simulink library "typhoonPatterns"  (R2017b)
settings: Solver=VariableStepAuto  StartTime=0.0  StopTime=10.0  RelTol=1e-3
undefined symbols (not defined in the file or in its folder): c_clamp, C_l, c_picoup_seq, crun_sp_ind, cst_sp_ind, f, f_picoup, f_sp_ind, fc, Jm, L, L1, L2, L_l, l_picoup_seq, La_DC, Ld, Lf_DC, Llr1_ind, Llr2_ind, Llr_ind, llrm_sp_ind, Lls_ind, llsa_sp_ind, llsm_sp_ind, Lm, Lq, n1, n2, nanm_sp_ind, pms, R, R1, R2, r_clamp, R_l, r_picoup_seq, Ra_DC, Rf_DC, Rm, Rr1_ind, Rr2_ind, Rr_ind, rrm_sp_ind, rrun_sp_ind, Rs, Rs_ind, rsa_sp_ind, rsm_sp_ind, rst_sp_ind
libraries: powerlib x282
(part 1 of 3)
settings Model: Creator=marco  LastModifiedBy=Marcos

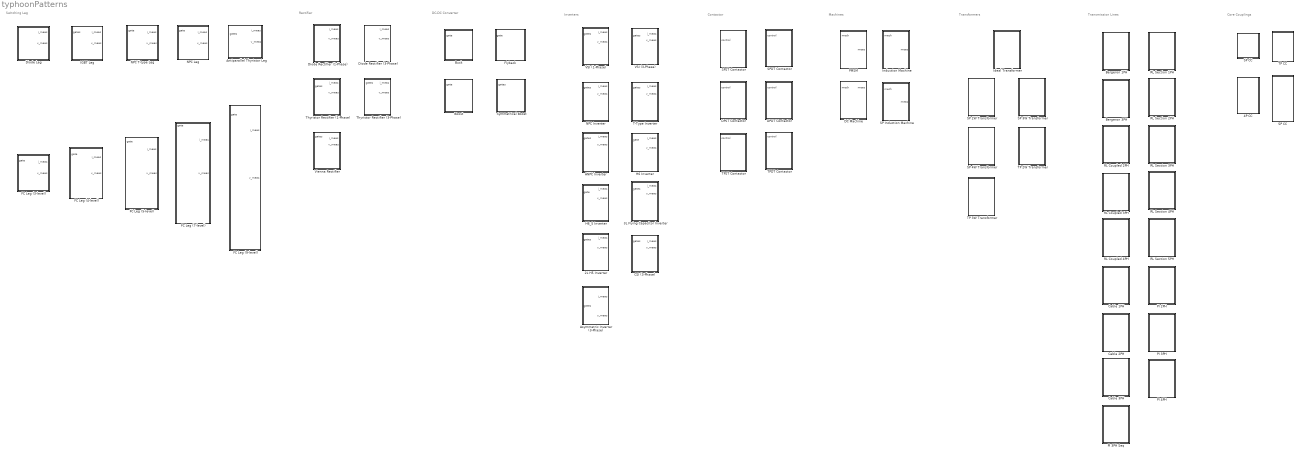
== system typhoonPatterns ==
  note: Rectifier
  note: Switching Leg
  note: DC-DC Converter
  note: Contactor
  note: Inverters
  note: Machines
  note: Transformers
  note: Transmission Lines
  note: Core Couplings
  2L H5 Inverter : Subsystem
  3L Flying Capacitor Inverter : Subsystem
  4P CC : Subsystem
  5P CC : Subsystem
  ANPC Inverter : Subsystem
  Antiparallel Thyristor Leg : Subsystem
  Asymmetric Inverter (3-Phase) : Subsystem
  Bergeron 1PH : Subsystem
  Bergeron 3PH : Subsystem
  Boost : Subsystem
  Buck : Subsystem
  CSI (3-Phase) : Subsystem
  Cable 1PH : Subsystem
  Cable 2PH : Subsystem
  Cable 3PH : Subsystem
  DC Machine : Subsystem
  DPDT Contactor : Subsystem
  DPST Contactor : Subsystem
  Diode Leg : Subsystem
  Diode Rectifier (1-Phase) : Subsystem
  Diode Rectifier (3-Phase) : Subsystem
  FC Leg (3-level) : Subsystem
  FC Leg (4-level) : Subsystem
  FC Leg (5-level) : Subsystem
  FC Leg (7-level) : Subsystem
  FC Leg (9-level) : Subsystem
  Flyback : Subsystem
  H6 Inverter : Subsystem
  H6_5 Inverter : Subsystem
  IGBT Leg : Subsystem
  Ideal Transformer : Subsystem
  Induction Machine : Subsystem
  NPC Inverter : Subsystem
  NPC Leg : Subsystem
  NPC T-type Leg : Subsystem
  PI 2PH : Subsystem
  PI 3PH : Subsystem
  PI 3PH Seq : Subsystem
  PI 4PH : Subsystem
  PMSM : Subsystem
  RL Coupled 2PH : Subsystem
  RL Coupled 3PH : Subsystem
  RL Coupled 4PH : Subsystem
  RL Section 1PH : Subsystem
  RL Section 2PH : Subsystem
  RL Section 3PH : Subsystem
  RL Section 4PH : Subsystem
  RL Section 5PH : Subsystem
  SP 2W Transformer : Subsystem
  SP 3W Transformer : Subsystem
  SP 4W Transformer : Subsystem
  SP CC : Subsystem
  SP Induction Machine : Subsystem
  SPDT Contactor : Subsystem
  SPST Contactor : Subsystem
  Symmetrical Boost : Subsystem
  T-Type Inverter : Subsystem
  TP 2W Transformer : Subsystem
  TP 3W Transformer : Subsystem
  TP CC : Subsystem
  TPDT Contactor : Subsystem
  TPST Contactor : Subsystem
  Thyristor Rectifier (1-Phase) : Subsystem
  Thyristor Rectifier (3-Phase) : Subsystem
  VSI (1-Phase) : Subsystem
  VSI (3-Phase) : Subsystem
  Vienna Rectifier : Subsystem

== system typhoonPatterns/2L H5 Inverter ==
  gates : Inport
  Bus Creator : BusCreator  Inputs=5
  Bus Creator1 : BusCreator  Inputs=5
  Demux{1..3,5..6} (5 alike) : Demux  Outputs=2
  Demux4 : Demux  Outputs=5
  S5 : powerlib/Power Electronics/IGBT//Diode  Ron=r_on  Rs=r_s  Cs=c_s  Measurements=on
  Selector_i : BusSelector  OutputSignals=i(Sa_top)  OutputAsBus=on
  Selector_v : BusSelector  OutputSignals=v(Sa_top)  OutputAsBus=on
  inv{1..5} (5 alike) : Logic  Commented=through  Operator=NOT  AllPortsSameDT=off  OutDataTypeStr=boolean
  sa_bot : powerlib/Power Electronics/IGBT//Diode  Ron=r_on  Rs=r_s  Cs=c_s  Measurements=on
  sa_top : powerlib/Power Electronics/IGBT//Diode  Ron=r_on  Rs=r_s  Cs=c_s  Measurements=on
  sb_bot : powerlib/Power Electronics/IGBT//Diode  Ron=r_on  Rs=r_s  Cs=c_s  Measurements=on
  sb_top : powerlib/Power Electronics/IGBT//Diode  Ron=r_on  Rs=r_s  Cs=c_s  Measurements=on
  A : PMIOPort  Port=1  Side=Right
  B : PMIOPort  Port=2  Side=Right
  DC+ : PMIOPort  Port=3  Side=Left
  DC- : PMIOPort  Port=4  Side=Left
  i_meas : Outport
  v_meas : Outport  Port=2
  wires:
  sb_top/1 -> [m_Sb_top]
  sa_top/1 -> [m_Sa_top]
  [Sb_top] -> sb_top/1
  sb_bot/1 -> [m_Sb_bot]
  [Sa_top] -> sa_top/1
  [Sb_bot] -> sb_bot/1
  sa_bot/1 -> [m_Sa_bot]
  [Sa_bot] -> sa_bot/1
  inv4/1 -> [Sb_bot]
  Demux4/4 -> inv4/1
  Demux4/2 -> inv2/1
  inv2/1 -> [Sa_bot]
  gates/1 -> Demux4/1
  inv3/1 -> [Sb_top]
  Demux4/3 -> inv3/1
  inv1/1 -> [Sa_top]
  Demux4/1 -> inv1/1
  Demux2/2 -> [v_Sa_bot]
  Demux1/2 -> [v_Sa_top]
  [v_Sa_top] -> Bus Creator1/1  "v(Sa_top)"
  [i_Sb_top] -> Bus Creator/3  "i(Sb_top)"
  [i_Sb_bot] -> Bus Creator/4  "i(Sb_bot)"
  Demux5/2 -> [v_Sb_bot]
  Bus Creator1/1 -> Selector_v/1
  Demux3/2 -> [v_Sb_top]
  [v_Sb_bot] -> Bus Creator1/4  "v(Sb_bot)"
  Demux5/1 -> [i_Sb_bot]
  Selector_v/1 -> v_meas/1
  [v_Sb_top] -> Bus Creator1/3  "v(Sb_top)"
  [m_Sb_bot] -> Demux5/1
  [m_Sa_bot] -> Demux2/1
  Demux1/1 -> [i_Sa_top]
  [m_Sa_top] -> Demux1/1
  Bus Creator/1 -> Selector_i/1
  [m_Sb_top] -> Demux3/1
  Demux2/1 -> [i_Sa_bot]
  Selector_i/1 -> i_meas/1
  Demux3/1 -> [i_Sb_top]
  [v_Sa_bot] -> Bus Creator1/2  "v(Sa_bot)"
  [i_Sa_bot] -> Bus Creator/2  "i(Sa_bot)"
  [i_Sa_top] -> Bus Creator/1  "i(Sa_top)"
  inv5/1 -> [S5]
  Demux4/5 -> inv5/1
  [S5] -> S5/1
  S5/1 -> [m_S5]
  [m_S5] -> Demux6/1
  Demux6/1 -> [i_S5]
  Demux6/2 -> [v_S5]
  [v_S5] -> Bus Creator1/5  "v(S5)"
  [i_S5] -> Bus Creator/5  "i(S5)"
  connections:
  sa_top/LConn1 -- sa_bot/RConn1 -- A/RConn1
  sb_top/LConn1 -- sb_bot/RConn1 -- B/RConn1
  sa_bot/LConn1 -- sb_bot/LConn1 -- DC-/RConn1
  sb_top/RConn1 -- S5/RConn1 -- sa_top/RConn1
  DC+/RConn1 -- S5/LConn1

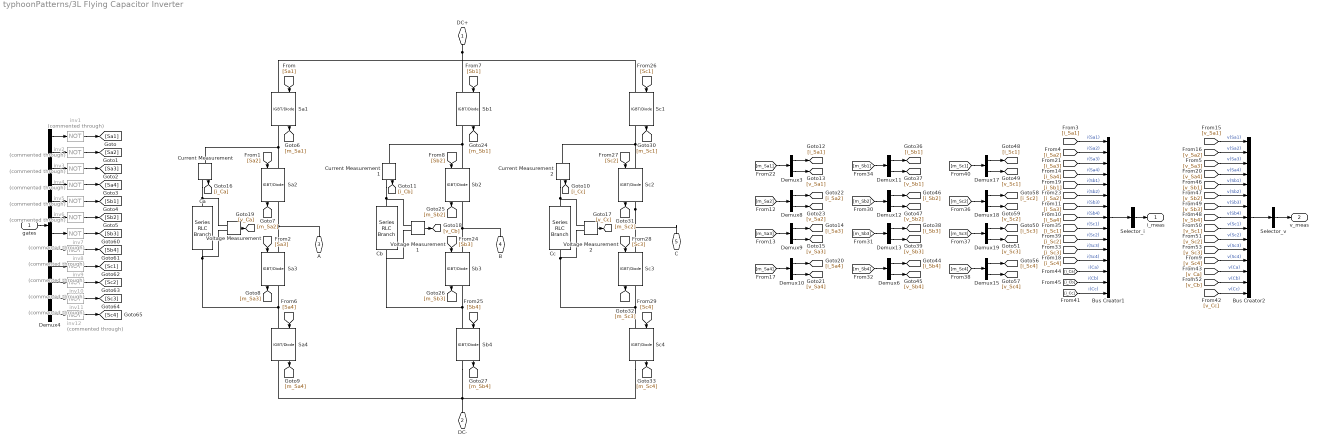
== system typhoonPatterns/3L Flying Capacitor Inverter ==
  gates : Inport
  Bus Creator1 : BusCreator  Inputs=15
  Bus Creator2 : BusCreator  Inputs=15
  Ca : powerlib/Elements/Series RLC Branch  LConnTagsString=__new0  RConnTagsString=__new0  BranchType=RC  Resistance=r_clamp  Inductance=1e-3  SetiL0=off  InitialCurrent=0  Capacitance=c_clamp  Setx0=on  InitialVoltage=v0_clamp  Measurements=None
  Cb : powerlib/Elements/Series RLC Branch  LConnTagsString=__new0  RConnTagsString=__new0  BranchType=RC  Resistance=r_clamp  Inductance=1e-3  SetiL0=off  InitialCurrent=0  Capacitance=c_clamp  Setx0=on  InitialVoltage=v0_clamp  Measurements=None
  Cc : powerlib/Elements/Series RLC Branch  LConnTagsString=__new0  RConnTagsString=__new0  BranchType=RC  Resistance=r_clamp  Inductance=1e-3  SetiL0=off  InitialCurrent=0  Capacitance=c_clamp  Setx0=on  InitialVoltage=v0_clamp  Measurements=None
  Current Measurement : powerlib/Measurements/Current Measurement  PhasorSimulation=off  OutputType=Complex  PSBequivalent=0
  Current Measurement1 : powerlib/Measurements/Current Measurement  PhasorSimulation=off  OutputType=Complex  PSBequivalent=0
  Current Measurement2 : powerlib/Measurements/Current Measurement  PhasorSimulation=off  OutputType=Complex  PSBequivalent=0
  Demux{3,6,8..13,15,17..19} (12 alike) : Demux  Outputs=2
  Demux4 : Demux  Outputs=12
  Sa{1..4} (4 alike) : powerlib/Power Electronics/IGBT//Diode  Ron=r_on  Rs=r_s  Cs=c_s  Measurements=on
  Sb{1..4} (4 alike) : powerlib/Power Electronics/IGBT//Diode  Ron=r_on  Rs=r_s  Cs=c_s  Measurements=on
  Sc{1..4} (4 alike) : powerlib/Power Electronics/IGBT//Diode  Ron=r_on  Rs=r_s  Cs=c_s  Measurements=on
  Selector_i : BusSelector  OutputSignals=i(Sa1)  OutputAsBus=on
  Selector_v : BusSelector  OutputSignals=v(Sa1)  OutputAsBus=on
  Voltage Measurement : powerlib/Measurements/Voltage Measurement  PhasorSimulation=off  OutputType=Complex  PSBequivalent=0
  Voltage Measurement1 : powerlib/Measurements/Voltage Measurement  PhasorSimulation=off  OutputType=Complex  PSBequivalent=0
  Voltage Measurement2 : powerlib/Measurements/Voltage Measurement  PhasorSimulation=off  OutputType=Complex  PSBequivalent=0
  inv{1..12} (12 alike) : Logic  Commented=through  Operator=NOT  AllPortsSameDT=off  OutDataTypeStr=boolean
  DC+ : PMIOPort  Port=1  Side=Left
  DC- : PMIOPort  Port=2  Side=Left
  A : PMIOPort  Port=3  Side=Right
  B : PMIOPort  Port=4  Side=Right
  C : PMIOPort  Port=5  Side=Right
  i_meas : Outport
  v_meas : Outport  Port=2
  wires:
  inv9/1 -> [Sc1]
  Demux4/7 -> inv7/1
  Demux4/11 -> inv11/1
  Demux4/9 -> inv9/1
  Demux4/8 -> inv8/1
  inv7/1 -> [Sb3]
  inv10/1 -> [Sc2]
  inv12/1 -> [Sc4]
  inv11/1 -> [Sc3]
  Demux4/10 -> inv10/1
  inv8/1 -> [Sb4]
  Demux4/12 -> inv12/1
  Demux17/1 -> [i_Sc1]
  Demux15/1 -> [i_Sc4]
  [m_Sc2] -> Demux18/1
  [m_Sc1] -> Demux17/1
  Demux19/1 -> [i_Sc3]
  Demux19/2 -> [v_Sc3]
  Demux17/2 -> [v_Sc1]
  Demux18/2 -> [v_Sc2]
  [m_Sc4] -> Demux15/1
  Demux15/2 -> [v_Sc4]
  Demux18/1 -> [i_Sc2]
  [m_Sc3] -> Demux19/1
  Demux11/1 -> [i_Sb1]
  Demux6/1 -> [i_Sb4]
  [m_Sb2] -> Demux12/1
  [m_Sb1] -> Demux11/1
  Demux13/1 -> [i_Sb3]
  Demux13/2 -> [v_Sb3]
  Demux11/2 -> [v_Sb1]
  Demux12/2 -> [v_Sb2]
  [m_Sb4] -> Demux6/1
  Demux6/2 -> [v_Sb4]
  Demux12/1 -> [i_Sb2]
  [m_Sb3] -> Demux13/1
  [Sc2] -> Sc2/1
  Sc1/1 -> [m_Sc1]
  Sc4/1 -> [m_Sc4]
  Sc2/1 -> [m_Sc2]
  [Sc1] -> Sc1/1
  Sc3/1 -> [m_Sc3]
  [Sc3] -> Sc3/1
  [Sc4] -> Sc4/1
  [Sb2] -> Sb2/1
  Sb1/1 -> [m_Sb1]
  Sb4/1 -> [m_Sb4]
  Sb2/1 -> [m_Sb2]
  [Sb1] -> Sb1/1
  Sb3/1 -> [m_Sb3]
  [Sb3] -> Sb3/1
  [Sb4] -> Sb4/1
  [Sa2] -> Sa2/1
  Sa1/1 -> [m_Sa1]
  Sa4/1 -> [m_Sa4]
  Sa2/1 -> [m_Sa2]
  [Sa1] -> Sa1/1
  Sa3/1 -> [m_Sa3]
  [Sa3] -> Sa3/1
  [Sa4] -> Sa4/1
  Selector_v/1 -> v_meas/1
  Demux3/1 -> [i_Sa1]
  Demux4/3 -> inv3/1
  [v_Sa4] -> Bus Creator2/4  "v(Sa4)"
  [v_Sa3] -> Bus Creator2/3  "v(Sa3)"
  inv4/1 -> [Sa4]
  [i_Sa4] -> Bus Creator1/4  "i(Sa4)"
  Demux3/2 -> [v_Sa1]
  inv2/1 -> [Sa2]
  inv1/1 -> [Sa1]
  inv5/1 -> [Sb1]
  inv3/1 -> [Sa3]
  gates/1 -> Demux4/1
  inv6/1 -> [Sb2]
  Demux4/1 -> inv1/1
  Demux4/6 -> inv6/1
  Demux8/1 -> [i_Sa2]
  Bus Creator2/1 -> Selector_v/1
  [i_Sa1] -> Bus Creator1/1  "i(Sa1)"
  Demux9/2 -> [v_Sa3]
  Demux9/1 -> [i_Sa3]
  [v_Sa1] -> Bus Creator2/1  "v(Sa1)"
  Demux8/2 -> [v_Sa2]
  [i_Sa3] -> Bus Creator1/3  "i(Sa3)"
  Demux4/5 -> inv5/1
  Demux10/2 -> [v_Sa4]
  Demux4/4 -> inv4/1
  [m_Sa2] -> Demux8/1
  [m_Sa3] -> Demux9/1
  [m_Sa4] -> Demux10/1
  Demux10/1 -> [i_Sa4]
  Bus Creator1/1 -> Selector_i/1
  [v_Sa2] -> Bus Creator2/2  "v(Sa2)"
  Selector_i/1 -> i_meas/1
  Demux4/2 -> inv2/1
  [m_Sa1] -> Demux3/1
  [i_Sa2] -> Bus Creator1/2  "i(Sa2)"
  Current Measurement/1 -> [i_Ca]
  Current Measurement1/1 -> [i_Cb]
  Current Measurement2/1 -> [i_Cc]
  Voltage Measurement/1 -> [v_Ca]
  Voltage Measurement2/1 -> [v_Cc]
  Voltage Measurement1/1 -> [v_Cb]
  [i_Cb] -> Bus Creator1/14  "i(Cb)"
  [i_Ca] -> Bus Creator1/13  "i(Ca)"
  [i_Cc] -> Bus Creator1/15  "i(Cc)"
  [i_Sa2] -> Bus Creator1/6  "i(Sb2)"
  [i_Sa3] -> Bus Creator1/7  "i(Sb3)"
  [i_Sb1] -> Bus Creator1/5  "i(Sb1)"
  [i_Sa4] -> Bus Creator1/8  "i(Sb4)"
  [i_Sc4] -> Bus Creator1/12  "i(Sc4)"
  [i_Sc3] -> Bus Creator1/11  "i(Sc3)"
  [i_Sc2] -> Bus Creator1/10  "i(Sc2)"
  [i_Sc1] -> Bus Creator1/9  "i(Sc1)"
  [v_Ca] -> Bus Creator2/13  "v(Ca)"
  [v_Cb] -> Bus Creator2/14  "v(Cb)"
  [v_Cc] -> Bus Creator2/15  "v(Cc)"
  [v_Sb3] -> Bus Creator2/7  "v(Sb3)"
  [v_Sb2] -> Bus Creator2/6  "v(Sb2)"
  [v_Sb1] -> Bus Creator2/5  "v(Sb1)"
  [v_Sb4] -> Bus Creator2/8  "v(Sb4)"
  [v_Sc3] -> Bus Creator2/11  "v(Sc3)"
  [v_Sc4] -> Bus Creator2/12  "v(Sc4)"
  [v_Sc2] -> Bus Creator2/10  "v(Sc2)"
  [v_Sc1] -> Bus Creator2/9  "v(Sc1)"
  connections:
  Sc2/LConn1 -- Current Measurement2/LConn1 -- Sc1/RConn1
  Sc4/LConn1 -- Voltage Measurement2/LConn2 -- Cc/RConn1 -- Sc3/RConn1
  Sc2/RConn1 -- Sc3/LConn1 -- C/RConn1
  Sb2/LConn1 -- Current Measurement1/LConn1 -- Sb1/RConn1
  Sb4/LConn1 -- Voltage Measurement1/LConn2 -- Cb/RConn1 -- Sb3/RConn1
  Sb3/LConn1 -- B/RConn1 -- Sb2/RConn1
  Sc4/RConn1 -- Sb4/RConn1 -- Sa4/RConn1 -- DC-/RConn1
  DC+/RConn1 -- Sb1/LConn1 -- Sc1/LConn1 -- Sa1/LConn1
  Ca/LConn1 -- Current Measurement/RConn1 -- Voltage Measurement/LConn1
  Sa4/LConn1 -- Voltage Measurement/LConn2 -- Ca/RConn1 -- Sa3/RConn1
  Sa3/LConn1 -- A/RConn1 -- Sa2/RConn1
  Sa2/LConn1 -- Current Measurement/LConn1 -- Sa1/RConn1
  Current Measurement1/RConn1 -- Voltage Measurement1/LConn1 -- Cb/LConn1
  Current Measurement2/RConn1 -- Voltage Measurement2/LConn1 -- Cc/LConn1

== system typhoonPatterns/4P CC ==
  a_in : PMIOPort  Port=1  Side=Left
  b_in : PMIOPort  Port=2  Side=Left
  a_out : PMIOPort  Port=3  Side=Right
  b_out : PMIOPort  Port=4  Side=Right
  c_in : PMIOPort  Port=5  Side=Left
  c_out : PMIOPort  Port=6  Side=Right
  d_in : PMIOPort  Port=7  Side=Left
  d_out : PMIOPort  Port=8  Side=Right
  connections:
  c_in/RConn1 -- c_out/RConn1
  b_in/RConn1 -- b_out/RConn1
  a_in/RConn1 -- a_out/RConn1
  d_in/RConn1 -- d_out/RConn1

== system typhoonPatterns/5P CC ==
  a_in : PMIOPort  Port=1  Side=Left
  b_in : PMIOPort  Port=2  Side=Left
  a_out : PMIOPort  Port=3  Side=Right
  b_out : PMIOPort  Port=4  Side=Right
  c_in : PMIOPort  Port=5  Side=Left
  c_out : PMIOPort  Port=6  Side=Right
  d_in : PMIOPort  Port=7  Side=Left
  d_out : PMIOPort  Port=8  Side=Right
  e_in : PMIOPort  Port=9  Side=Left
  e_out : PMIOPort  Port=10  Side=Right
  connections:
  c_in/RConn1 -- c_out/RConn1
  a_in/RConn1 -- a_out/RConn1
  b_in/RConn1 -- b_out/RConn1
  d_in/RConn1 -- d_out/RConn1
  e_in/RConn1 -- e_out/RConn1

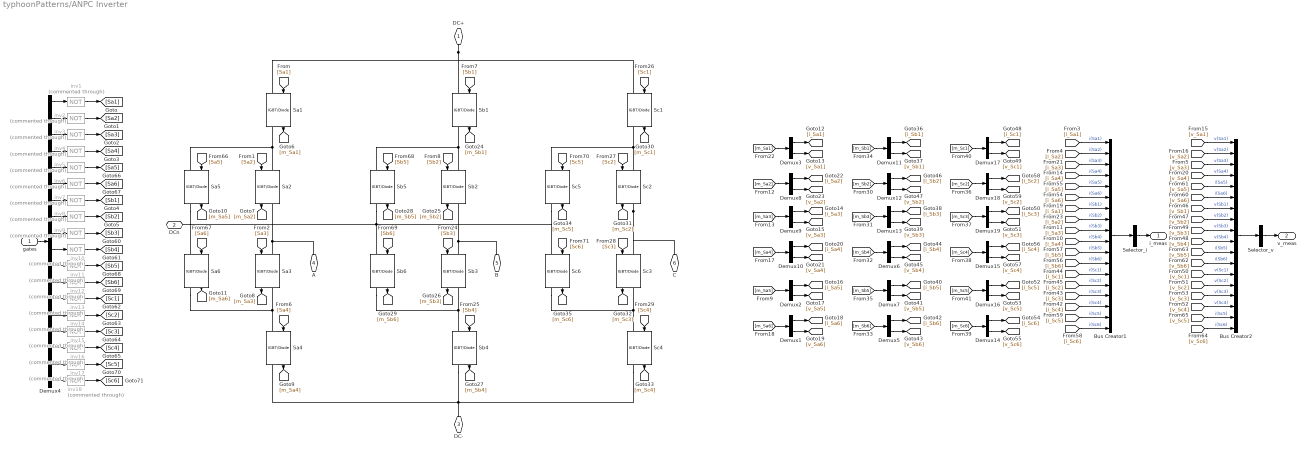
== system typhoonPatterns/ANPC Inverter ==
  gates : Inport
  Bus Creator1 : BusCreator  Inputs=18
  Bus Creator2 : BusCreator  Inputs=18
  Demux{1..3,5..19} (18 alike) : Demux  Outputs=2
  Demux4 : Demux  Outputs=18
  Sa{1..6} (6 alike) : powerlib/Power Electronics/IGBT//Diode  Ron=r_on  Rs=r_s  Cs=c_s  Measurements=on
  Sb{1..6} (6 alike) : powerlib/Power Electronics/IGBT//Diode  Ron=r_on  Rs=r_s  Cs=c_s  Measurements=on
  Sc{1..6} (6 alike) : powerlib/Power Electronics/IGBT//Diode  Ron=r_on  Rs=r_s  Cs=c_s  Measurements=on
  Selector_i : BusSelector  OutputSignals=i(Sa1)  OutputAsBus=on
  Selector_v : BusSelector  OutputSignals=v(Sa1)  OutputAsBus=on
  inv{1..18} (18 alike) : Logic  Commented=through  Operator=NOT  AllPortsSameDT=off  OutDataTypeStr=boolean
  DC+ : PMIOPort  Port=1  Side=Left
  DCn : PMIOPort  Port=2  Side=Left
  DC- : PMIOPort  Port=3  Side=Left
  A : PMIOPort  Port=4  Side=Right
  B : PMIOPort  Port=5  Side=Right
  C : PMIOPort  Port=6  Side=Right
  i_meas : Outport
  v_meas : Outport  Port=2
  wires:
  [v_Sa5] -> Bus Creator2/5  "i(Sa5)"
  [v_Sb6] -> Bus Creator2/12  "i(Sb6)"
  [v_Sc5] -> Bus Creator2/17  "i(Sc5)"
  [v_Sc6] -> Bus Creator2/18  "i(Sc6)"
  [v_Sb5] -> Bus Creator2/11  "i(Sb5)"
  [v_Sa6] -> Bus Creator2/6  "i(Sa6)"
  [i_Sc6] -> Bus Creator1/18  "i(Sc6)"
  [i_Sc5] -> Bus Creator1/17  "i(Sc5)"
  [i_Sb6] -> Bus Creator1/12  "i(Sb6)"
  [i_Sb5] -> Bus Creator1/11  "i(Sb5)"
  [i_Sa5] -> Bus Creator1/5  "i(Sa5)"
  [i_Sa6] -> Bus Creator1/6  "i(Sa6)"
  [v_Sb1] -> Bus Creator2/7  "v(Sb1)"
  [v_Sb2] -> Bus Creator2/8  "v(Sb2)"
  [v_Sb3] -> Bus Creator2/9  "v(Sb3)"
  [v_Sb4] -> Bus Creator2/10  "v(Sb4)"
  [v_Sc2] -> Bus Creator2/14  "v(Sc2)"
  [v_Sc4] -> Bus Creator2/16  "v(Sc4)"
  [v_Sc3] -> Bus Creator2/15  "v(Sc3)"
  [v_Sc1] -> Bus Creator2/13  "v(Sc1)"
  [i_Sa4] -> Bus Creator1/10  "i(Sb4)"
  [i_Sa3] -> Bus Creator1/9  "i(Sb3)"
  [i_Sa2] -> Bus Creator1/8  "i(Sb2)"
  [i_Sa1] -> Bus Creator1/7  "i(Sb1)"
  [i_Sc1] -> Bus Creator1/13  "i(Sc1)"
  [i_Sc2] -> Bus Creator1/14  "i(Sc2)"
  [i_Sc4] -> Bus Creator1/16  "i(Sc4)"
  [i_Sc3] -> Bus Creator1/15  "i(Sc3)"
  Demux4/7 -> inv7/1
  Demux4/11 -> inv11/1
  Demux4/9 -> inv9/1
  Demux4/8 -> inv8/1
  Demux4/10 -> inv10/1
  Demux4/12 -> inv12/1
  Demux17/1 -> [i_Sc1]
  Demux15/1 -> [i_Sc4]
  [m_Sc2] -> Demux18/1
  [m_Sc1] -> Demux17/1
  Demux19/1 -> [i_Sc3]
  [m_Sc6] -> Demux14/1
  Demux16/2 -> [v_Sc5]
  Demux19/2 -> [v_Sc3]
  Demux16/1 -> [i_Sc5]
  Demux17/2 -> [v_Sc1]
  Demux18/2 -> [v_Sc2]
  [m_Sc4] -> Demux15/1
  Demux15/2 -> [v_Sc4]
  Demux14/2 -> [v_Sc6]
  Demux18/1 -> [i_Sc2]
  [m_Sc5] -> Demux16/1
  Demux14/1 -> [i_Sc6]
  [m_Sc3] -> Demux19/1
  Demux11/1 -> [i_Sb1]
  Demux6/1 -> [i_Sb4]
  [m_Sb2] -> Demux12/1
  [m_Sb1] -> Demux11/1
  Demux13/1 -> [i_Sb3]
  [m_Sb6] -> Demux5/1
  Demux7/2 -> [v_Sb5]
  Demux13/2 -> [v_Sb3]
  Demux7/1 -> [i_Sb5]
  Demux11/2 -> [v_Sb1]
  Demux12/2 -> [v_Sb2]
  [m_Sb4] -> Demux6/1
  Demux6/2 -> [v_Sb4]
  Demux5/2 -> [v_Sb6]
  Demux12/1 -> [i_Sb2]
  [m_Sb5] -> Demux7/1
  Demux5/1 -> [i_Sb6]
  [m_Sb3] -> Demux13/1
  [Sc2] -> Sc2/1
  Sc1/1 -> [m_Sc1]
  Sc4/1 -> [m_Sc4]
  Sc2/1 -> [m_Sc2]
  [Sc1] -> Sc1/1
  Sc3/1 -> [m_Sc3]
  [Sc3] -> Sc3/1
  [Sc4] -> Sc4/1
  [Sb2] -> Sb2/1
  Sb1/1 -> [m_Sb1]
  Sb4/1 -> [m_Sb4]
  Sb2/1 -> [m_Sb2]
  [Sb1] -> Sb1/1
  Sb3/1 -> [m_Sb3]
  [Sb3] -> Sb3/1
  [Sb4] -> Sb4/1
  [Sa2] -> Sa2/1
  Sa1/1 -> [m_Sa1]
  Sa4/1 -> [m_Sa4]
  Sa2/1 -> [m_Sa2]
  [Sa1] -> Sa1/1
  Sa3/1 -> [m_Sa3]
  [Sa3] -> Sa3/1
  [Sa4] -> Sa4/1
  Selector_v/1 -> v_meas/1
  Demux1/1 -> [i_Sa6]
  Demux3/1 -> [i_Sa1]
  Demux4/3 -> inv3/1
  [v_Sa4] -> Bus Creator2/4  "v(Sa4)"
  [v_Sa3] -> Bus Creator2/3  "v(Sa3)"
  inv4/1 -> [Sa4]
  [i_Sa4] -> Bus Creator1/4  "i(Sa4)"
  Demux3/2 -> [v_Sa1]
  inv2/1 -> [Sa2]
  Demux1/2 -> [v_Sa6]
  inv1/1 -> [Sa1]
  inv3/1 -> [Sa3]
  gates/1 -> Demux4/1
  Demux4/1 -> inv1/1
  Demux4/6 -> inv6/1
  Demux8/1 -> [i_Sa2]
  Bus Creator2/1 -> Selector_v/1
  [i_Sa1] -> Bus Creator1/1  "i(Sa1)"
  Demux9/2 -> [v_Sa3]
  Demux9/1 -> [i_Sa3]
  [v_Sa1] -> Bus Creator2/1  "v(Sa1)"
  Demux8/2 -> [v_Sa2]
  [i_Sa3] -> Bus Creator1/3  "i(Sa3)"
  Demux4/5 -> inv5/1
  Demux10/2 -> [v_Sa4]
  Demux4/4 -> inv4/1
  [m_Sa2] -> Demux8/1
  Demux2/1 -> [i_Sa5]
  [m_Sa3] -> Demux9/1
  [m_Sa4] -> Demux10/1
  Demux10/1 -> [i_Sa4]
  [m_Sa5] -> Demux2/1
  Demux2/2 -> [v_Sa5]
  Bus Creator1/1 -> Selector_i/1
  [v_Sa2] -> Bus Creator2/2  "v(Sa2)"
  [m_Sa6] -> Demux1/1
  Selector_i/1 -> i_meas/1
  Demux4/2 -> inv2/1
  [m_Sa1] -> Demux3/1
  [i_Sa2] -> Bus Creator1/2  "i(Sa2)"
  Sa5/1 -> [m_Sa5]
  Sa6/1 -> [m_Sa6]
  Sc6/1 -> [m_Sc6]
  Sc5/1 -> [m_Sc5]
  Sb5/1 -> [m_Sb5]
  Sb6/1 -> [m_Sb6]
  Demux4/13 -> inv13/1
  Demux4/14 -> inv14/1
  Demux4/15 -> inv15/1
  Demux4/16 -> inv16/1
  Demux4/17 -> inv17/1
  Demux4/18 -> inv18/1
  inv16/1 -> [Sc4]
  inv14/1 -> [Sc2]
  inv15/1 -> [Sc3]
  inv13/1 -> [Sc1]
  inv8/1 -> [Sb2]
  inv10/1 -> [Sb4]
  inv9/1 -> [Sb3]
  inv7/1 -> [Sb1]
  inv5/1 -> [Sa5]
  inv6/1 -> [Sa6]
  [Sa5] -> Sa5/1
  [Sa6] -> Sa6/1
  inv11/1 -> [Sb5]
  inv12/1 -> [Sb6]
  inv18/1 -> [Sc6]
  inv17/1 -> [Sc5]
  [Sc6] -> Sc6/1
  [Sc5] -> Sc5/1
  [Sb5] -> Sb5/1
  [Sb6] -> Sb6/1
  connections:
  Sc2/LConn1 -- Sc5/LConn1 -- Sc1/RConn1
  Sc4/LConn1 -- Sc6/RConn1 -- Sc3/RConn1
  Sc2/RConn1 -- Sc3/LConn1 -- C/RConn1
  Sc6/LConn1 -- Sc5/RConn1 -- DCn/RConn1 -- Sa6/LConn1 -- Sa5/RConn1 -- Sb6/LConn1 -- Sb5/RConn1
  Sb2/LConn1 -- Sb5/LConn1 -- Sb1/RConn1
  Sb4/LConn1 -- Sb6/RConn1 -- Sb3/RConn1
  Sb3/LConn1 -- Sb2/RConn1 -- B/RConn1
  Sc4/RConn1 -- Sb4/RConn1 -- Sa4/RConn1 -- DC-/RConn1
  DC+/RConn1 -- Sb1/LConn1 -- Sc1/LConn1 -- Sa1/LConn1
  Sa2/LConn1 -- Sa5/LConn1 -- Sa1/RConn1
  Sa4/LConn1 -- Sa6/RConn1 -- Sa3/RConn1
  Sa3/LConn1 -- Sa2/RConn1 -- A/RConn1

== system typhoonPatterns/Antiparallel Thyristor Leg ==
  gates : Inport
  Bus Creator : BusCreator  Inputs=2
  Bus Creator1 : BusCreator  Inputs=2
  Demux1 : Demux  Outputs=2
  Demux2 : Demux  Outputs=2
  Demux4 : Demux  Outputs=2
  S1 (T1) : powerlib/Power Electronics/Thyristor  Ron=r_on  Lon=0  Vf=v_f  IC=0  Rs=r_s  Cs=c_s  Measurements=on
  S2 (T2) : powerlib/Power Electronics/Thyristor  Ron=r_on  Lon=0  Vf=v_f  IC=0  Rs=r_s  Cs=c_s  Measurements=on
  Selector_i : BusSelector  OutputSignals=i(T1)  OutputAsBus=on
  Selector_v : BusSelector  OutputSignals=v(T1)  OutputAsBus=on
  inv1 : Logic  Commented=through  Operator=NOT  AllPortsSameDT=off  OutDataTypeStr=boolean
  inv2 : Logic  Commented=through  Operator=NOT  AllPortsSameDT=off  OutDataTypeStr=boolean
  Phase + : PMIOPort  Port=1  Side=Left
  Phase - : PMIOPort  Port=2  Side=Right
  i_meas : Outport
  v_meas : Outport  Port=2
  wires:
  [i_S1] -> Bus Creator/1  "i(T1)"
  Demux4/1 -> inv1/1
  [i_S2] -> Bus Creator/2  "i(T2)"
  Demux4/2 -> inv2/1
  Bus Creator1/1 -> Selector_v/1
  inv1/1 -> [S1]
  Selector_v/1 -> v_meas/1
  Demux2/1 -> [i_S2]
  Demux2/2 -> [v_S2]
  Selector_i/1 -> i_meas/1
  [v_S2] -> Bus Creator1/2  "v(T2)"
  Bus Creator/1 -> Selector_i/1
  gates/1 -> Demux4/1
  inv2/1 -> [S2]
  Demux1/2 -> [v_S1]
  Demux1/1 -> [i_S1]
  [v_S1] -> Bus Creator1/1  "v(T1)"
  [m_S2] -> Demux2/1
  [m_S1] -> Demux1/1
  S2 (T2)/1 -> [m_S2]
  S1 (T1)/1 -> [m_S1]
  [S1] -> S1 (T1)/1
  [S2] -> S2 (T2)/1
  connections:
  S2 (T2)/LConn1 -- S1 (T1)/RConn1 -- Phase -/RConn1
  S2 (T2)/RConn1 -- S1 (T1)/LConn1 -- Phase +/RConn1

== system typhoonPatterns/Asymmetric Inverter (3-Phase) ==
  gates : Inport
  Bus Creator1 : BusCreator  Inputs=6
  Bus Creator2 : BusCreator  Inputs=6
  Demux{1..3,8..10} (6 alike) : Demux  Outputs=2
  Demux4 : Demux  Outputs=6
  Selector_i : BusSelector  OutputSignals=i(Sa_top)  OutputAsBus=on
  Selector_v : BusSelector  OutputSignals=v(Sa_top)  OutputAsBus=on
  inv{1..6} (6 alike) : Logic  Commented=through  Operator=NOT  AllPortsSameDT=off  OutDataTypeStr=boolean
  i_meas : Outport
  v_meas : Outport  Port=2
  wires:
  [v_Sc_top] -> Bus Creator2/5  "v(Sc_top)"
  [v_Sc_bot] -> Bus Creator2/6  "v(Sc_bot)"
  Demux1/2 -> [v_Sc_bot]
  [m_Sc_bot] -> Demux1/1
  [m_Sa_bot] -> Demux10/1
  [i_Sc_bot] -> Bus Creator1/5  "i(Sc_top)"
  [i_Sc_bot] -> Bus Creator1/6  "i(Sc_bot)"
  Demux1/1 -> [i_Sc_bot]
  [m_Sb_top] -> Demux9/1
  [m_Sc_top] -> Demux2/1
  Demux2/1 -> [i_Sc_top]
  [v_Sa_top] -> Bus Creator2/1  "v(Sa_top)"
  Demux2/2 -> [v_Sc_top]
  [i_Sa_bot] -> Bus Creator1/2  "i(Sa_bot)"
  [i_Sb_top] -> Bus Creator1/3  "i(Sb_top)"
  Demux8/2 -> [v_Sa_bot]
  Demux3/2 -> [v_Sa_top]
  Demux9/2 -> [v_Sb_top]
  Demux8/1 -> [i_Sa_bot]
  Demux10/1 -> [i_Sb_bot]
  [v_Sb_top] -> Bus Creator2/3  "v(Sb_top)"
  [i_Sb_bot] -> Bus Creator1/4  "i(Sb_bot)"
  Demux10/2 -> [v_Sb_bot]
  Selector_v/1 -> v_meas/1
  Selector_i/1 -> i_meas/1
  Bus Creator2/1 -> Selector_v/1
  [v_Sb_bot] -> Bus Creator2/4  "v(Sb_bot)"
  [m_Sa_top] -> Demux3/1
  Demux9/1 -> [i_Sb_top]
  [m_Sa_bot] -> Demux8/1
  Demux3/1 -> [i_Sa_top]
  [i_Sa_top] -> Bus Creator1/1  "i(Sa_top)"
  Bus Creator1/1 -> Selector_i/1
  [v_Sa_bot] -> Bus Creator2/2  "v(Sa_bot)"
  Demux4/4 -> inv4/1
  inv5/1 -> [Sc_top]
  inv4/1 -> [Sb_bot]
  Demux4/6 -> inv6/1
  inv6/1 -> [Sc_bot]
  Demux4/5 -> inv5/1
  gates/1 -> Demux4/1
  Demux4/3 -> inv3/1
  Demux4/1 -> inv1/1
  inv1/1 -> [Sa_top]
  Demux4/2 -> inv2/1
  inv3/1 -> [Sb_top]
  inv2/1 -> [Sa_bot]

== system typhoonPatterns/Bergeron 1PH ==
  Distributed Parameters Line : powerlib/Elements/Distributed Parameters Line  Phases=2  Frequency=f  Resistance=R_l  Inductance=L_l  Capacitance=C_l  Length=length  x1=[0 0 0 0; 0.0001244 0 0 0; 0.0002488 0 0 0; 0.0003733 0 0 0; 0.0004977 0 0 0; 0.0006221 0 0 0]  x2=[0 0 0 0; 0.0001244 0 0 0; 0.0002488 0 0 0; 0.0003733 0 0 0; 0.0004977 0 0 0; 0.0006221 0 0 0]  x3=[0 0 0 0; 0.0001244 0 0 0; 0.0002488 0 0 0; 0.0003733 0 0 0; 0.0004977 0 0 0; 0.0006221 0 0 0]  x4=[0 0 0 0; 0.0001244 0 0 0; 0.0002488 0 0 0; 0.0003733 0 0 0; 0.0004977 0 0 0; 0.0006221 0 0 0]  x5=0  V1=ones(3,3)  V2=ones(3,3)  I1=ones(3,3)  I2=ones(3,3)  nHarmo=1  Measurements=None
      settings: SourceProductName=Simscape Power Systems
  a_in : PMIOPort  Port=1  Side=Left
  a_out : PMIOPort  Port=2  Side=Right
  b_in : PMIOPort  Port=3  Side=Left
  b_out : PMIOPort  Port=4  Side=Right
  connections:
  b_out/RConn1 -- Distributed Parameters Line/RConn2
  Distributed Parameters Line/RConn1 -- a_out/RConn1
  Distributed Parameters Line/LConn1 -- a_in/RConn1
  b_in/RConn1 -- Distributed Parameters Line/LConn2

== system typhoonPatterns/Bergeron 3PH ==
  Distributed Parameters Line : powerlib/Elements/Distributed Parameters Line  Phases=3  Frequency=f  Resistance=R_l  Inductance=L_l  Capacitance=C_l  Length=length  x1=[0 0 0 0; 0.0001244 0 0 0; 0.0002488 0 0 0; 0.0003733 0 0 0; 0.0004977 0 0 0; 0.0006221 0 0 0]  x2=[0 0 0 0; 0.0001244 0 0 0; 0.0002488 0 0 0; 0.0003733 0 0 0; 0.0004977 0 0 0; 0.0006221 0 0 0]  x3=[0 0 0 0; 0.0001244 0 0 0; 0.0002488 0 0 0; 0.0003733 0 0 0; 0.0004977 0 0 0; 0.0006221 0 0 0]  x4=[0 0 0 0; 0.0001244 0 0 0; 0.0002488 0 0 0; 0.0003733 0 0 0; 0.0004977 0 0 0; 0.0006221 0 0 0]  x5=0  V1=ones(3,3)  V2=ones(3,3)  I1=ones(3,3)  I2=ones(3,3)  nHarmo=1  Measurements=None
      settings: SourceProductName=Simscape Power Systems
  a_in : PMIOPort  Port=1  Side=Left
  a_out : PMIOPort  Port=2  Side=Right
  b_in : PMIOPort  Port=3  Side=Left
  b_out : PMIOPort  Port=4  Side=Right
  c_in : PMIOPort  Port=5  Side=Left
  c_out : PMIOPort  Port=6  Side=Right
  connections:
  Distributed Parameters Line/RConn3 -- c_out/RConn1
  Distributed Parameters Line/LConn3 -- c_in/RConn1
  Distributed Parameters Line/LConn2 -- b_in/RConn1
  Distributed Parameters Line/LConn1 -- a_in/RConn1
  Distributed Parameters Line/RConn1 -- a_out/RConn1
  Distributed Parameters Line/RConn2 -- b_out/RConn1

== system typhoonPatterns/Boost ==
  gate : Inport
  Boost Converter : powerlib/Power Electronics/Boost Converter  ModelType=Switching devices  Ron=r_on  Rs=r_s  Cs=c_s  Vforward=[0, 0]  Ron_Diode=1e-3  Rs_Diode=1e6  Cs_Diode=inf  Vf_Diode=1e-3  Rs_CurrentSource=inf
      settings: SourceProductName=Simscape Power Systems  SourceProductBaseCode=PS
  inv1 : Logic  Commented=through  Operator=NOT  AllPortsSameDT=off  OutDataTypeStr=boolean
  In+ : PMIOPort  Port=1  Side=Left
  In- : PMIOPort  Port=2  Side=Left
  Out+ : PMIOPort  Port=3  Side=Right
  Out- : PMIOPort  Port=4  Side=Right
  wires:
  inv1/1 -> Boost Converter/1
  gate/1 -> inv1/1
  connections:
  In+/RConn1 -- Boost Converter/RConn1
  In-/RConn1 -- Out+/RConn1 -- Boost Converter/RConn2
  Out-/RConn1 -- Boost Converter/LConn1

== system typhoonPatterns/Buck ==
  gate : Inport
  Buck Converter : powerlib/Power Electronics/Buck Converter  ModelType=Switching devices  Ron=r_on  Rs=r_s  Cs=c_s  Vforward=[0,0]  Ron_Diode=1e-3  Rs_Diode=1e6  Cs_Diode=inf  Vf_Diode=1e-3  Rs_CurrentSource=inf
      settings: SourceProductName=Simscape Power Systems  SourceProductBaseCode=PS
  inv1 : Logic  Commented=through  Operator=NOT  AllPortsSameDT=off  OutDataTypeStr=boolean
  In+ : PMIOPort  Port=1  Side=Left
  In- : PMIOPort  Port=2  Side=Left
  Out+ : PMIOPort  Port=3  Side=Right
  Out- : PMIOPort  Port=4  Side=Right
  wires:
  inv1/1 -> Buck Converter/1
  gate/1 -> inv1/1
  connections:
  In+/RConn1 -- Buck Converter/RConn1
  In-/RConn1 -- Out-/RConn1 -- Buck Converter/RConn2
  Out+/RConn1 -- Buck Converter/LConn1

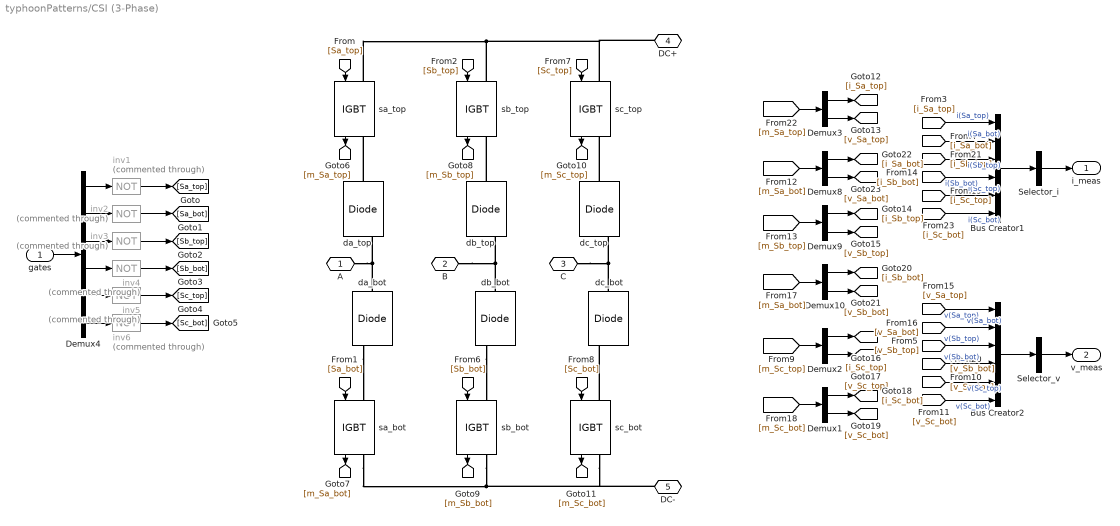
== system typhoonPatterns/CSI (3-Phase) ==
  gates : Inport
  Bus Creator1 : BusCreator  Inputs=6
  Bus Creator2 : BusCreator  Inputs=6
  Demux{1..3,8..10} (6 alike) : Demux  Outputs=2
  Demux4 : Demux  Outputs=6
  Selector_i : BusSelector  OutputSignals=i(Sa_top)  OutputAsBus=on
  Selector_v : BusSelector  OutputSignals=v(Sa_top)  OutputAsBus=on
  da_bot : powerlib/Power Electronics/Diode  Ron=r_on  Lon=0  Vf=v_f  IC=0  UseSnubber=0  Rs=r_s  Cs=c_s  Measurements=on
  da_top : powerlib/Power Electronics/Diode  Ron=r_on  Lon=0  Vf=v_f  IC=0  UseSnubber=0  Rs=r_s  Cs=c_s  Measurements=on
  db_bot : powerlib/Power Electronics/Diode  Ron=r_on  Lon=0  Vf=v_f  IC=0  UseSnubber=0  Rs=r_s  Cs=c_s  Measurements=on
  db_top : powerlib/Power Electronics/Diode  Ron=r_on  Lon=0  Vf=v_f  IC=0  UseSnubber=0  Rs=r_s  Cs=c_s  Measurements=on
  dc_bot : powerlib/Power Electronics/Diode  Ron=r_on  Lon=0  Vf=v_f  IC=0  UseSnubber=0  Rs=r_s  Cs=c_s  Measurements=on
  dc_top : powerlib/Power Electronics/Diode  Ron=r_on  Lon=0  Vf=v_f  IC=0  UseSnubber=0  Rs=r_s  Cs=c_s  Measurements=on
  inv{1..6} (6 alike) : Logic  Commented=through  Operator=NOT  AllPortsSameDT=off  OutDataTypeStr=boolean
  sa_bot : powerlib/Power Electronics/IGBT  Ron=r_on  Lon=0  Vf=v_f  Tf=1e-6  Tt=2e-6  IC=0  Rs=r_s  Cs=c_s  Measurements=on
  sa_top : powerlib/Power Electronics/IGBT  Ron=r_on  Lon=0  Vf=v_f  Tf=1e-6  Tt=2e-6  IC=0  Rs=r_s  Cs=c_s  Measurements=on
  sb_bot : powerlib/Power Electronics/IGBT  Ron=r_on  Lon=0  Vf=v_f  Tf=1e-6  Tt=2e-6  IC=0  Rs=r_s  Cs=c_s  Measurements=on
  sb_top : powerlib/Power Electronics/IGBT  Ron=r_on  Lon=0  Vf=v_f  Tf=1e-6  Tt=2e-6  IC=0  Rs=r_s  Cs=c_s  Measurements=on
  sc_bot : powerlib/Power Electronics/IGBT  Ron=r_on  Lon=0  Vf=v_f  Tf=1e-6  Tt=2e-6  IC=0  Rs=r_s  Cs=c_s  Measurements=on
  sc_top : powerlib/Power Electronics/IGBT  Ron=r_on  Lon=0  Vf=v_f  Tf=1e-6  Tt=2e-6  IC=0  Rs=r_s  Cs=c_s  Measurements=on
  A : PMIOPort  Port=1  Side=Right
  B : PMIOPort  Port=2  Side=Right
  C : PMIOPort  Port=3  Side=Right
  DC+ : PMIOPort  Port=4  Side=Left
  DC- : PMIOPort  Port=5  Side=Left
  i_meas : Outport
  v_meas : Outport  Port=2
  wires:
  [v_Sc_top] -> Bus Creator2/5  "v(Sc_top)"
  [v_Sc_bot] -> Bus Creator2/6  "v(Sc_bot)"
  Demux1/2 -> [v_Sc_bot]
  [m_Sc_bot] -> Demux1/1
  [m_Sa_bot] -> Demux10/1
  [i_Sc_top] -> Bus Creator1/5  "i(Sc_top)"
  [i_Sc_bot] -> Bus Creator1/6  "i(Sc_bot)"
  Demux1/1 -> [i_Sc_bot]
  [m_Sb_top] -> Demux9/1
  [m_Sc_top] -> Demux2/1
  Demux2/1 -> [i_Sc_top]
  [v_Sa_top] -> Bus Creator2/1  "v(Sa_top)"
  Demux2/2 -> [v_Sc_top]
  [i_Sa_bot] -> Bus Creator1/2  "i(Sa_bot)"
  [i_Sb_top] -> Bus Creator1/3  "i(Sb_top)"
  Demux8/2 -> [v_Sa_bot]
  Demux3/2 -> [v_Sa_top]
  Demux9/2 -> [v_Sb_top]
  Demux8/1 -> [i_Sa_bot]
  Demux10/1 -> [i_Sb_bot]
  [v_Sb_top] -> Bus Creator2/3  "v(Sb_top)"
  [i_Sb_bot] -> Bus Creator1/4  "i(Sb_bot)"
  Demux10/2 -> [v_Sb_bot]
  Selector_v/1 -> v_meas/1
  Selector_i/1 -> i_meas/1
  Bus Creator2/1 -> Selector_v/1
  [v_Sb_bot] -> Bus Creator2/4  "v(Sb_bot)"
  [m_Sa_top] -> Demux3/1
  Demux9/1 -> [i_Sb_top]
  [m_Sa_bot] -> Demux8/1
  Demux3/1 -> [i_Sa_top]
  [i_Sa_top] -> Bus Creator1/1  "i(Sa_top)"
  Bus Creator1/1 -> Selector_i/1
  [v_Sa_bot] -> Bus Creator2/2  "v(Sa_bot)"
  Demux4/4 -> inv4/1
  inv5/1 -> [Sc_top]
  inv4/1 -> [Sb_bot]
  Demux4/6 -> inv6/1
  inv6/1 -> [Sc_bot]
  Demux4/5 -> inv5/1
  gates/1 -> Demux4/1
  Demux4/3 -> inv3/1
  Demux4/1 -> inv1/1
  inv1/1 -> [Sa_top]
  Demux4/2 -> inv2/1
  inv3/1 -> [Sb_top]
  inv2/1 -> [Sa_bot]
  sa_top/1 -> [m_Sa_top]
  [Sa_top] -> sa_top/1
  sb_top/1 -> [m_Sb_top]
  sc_top/1 -> [m_Sc_top]
  sa_bot/1 -> [m_Sa_bot]
  sb_bot/1 -> [m_Sb_bot]
  sc_bot/1 -> [m_Sc_bot]
  [Sc_bot] -> sc_bot/1
  [Sb_bot] -> sb_bot/1
  [Sa_bot] -> sa_bot/1
  [Sb_top] -> sb_top/1
  [Sc_top] -> sc_top/1
  connections:
  sc_top/LConn1 -- DC+/RConn1 -- sb_top/LConn1 -- sa_top/LConn1
  sc_bot/RConn1 -- DC-/RConn1 -- sb_bot/RConn1 -- sa_bot/RConn1
  da_top/LConn1 -- sa_top/RConn1
  da_bot/RConn1 -- sa_bot/LConn1
  da_bot/LConn1 -- A/RConn1 -- da_top/RConn1
  db_bot/LConn1 -- B/RConn1 -- db_top/RConn1
  dc_bot/LConn1 -- C/RConn1 -- dc_top/RConn1
  db_bot/RConn1 -- sb_bot/LConn1
  sc_bot/LConn1 -- dc_bot/RConn1
  dc_top/LConn1 -- sc_top/RConn1
  db_top/LConn1 -- sb_top/RConn1

== system typhoonPatterns/Cable 1PH ==
  RL1 : powerlib/Elements/Series RLC Branch  LConnTagsString=__new0  RConnTagsString=__new0  BranchType=RL  Resistance=R  Inductance=L  SetiL0=off  InitialCurrent=0  Capacitance=1e-6  Setx0=off  InitialVoltage=0  Measurements=None
  a_in : PMIOPort  Port=1  Side=Left
  a_out : PMIOPort  Port=2  Side=Right
  connections:
  a_out/RConn1 -- RL1/RConn1
  a_in/RConn1 -- RL1/LConn1

== system typhoonPatterns/Cable 2PH ==
  RL1 : powerlib/Elements/Series RLC Branch  LConnTagsString=__new0  RConnTagsString=__new0  BranchType=RL  Resistance=R  Inductance=L  SetiL0=off  InitialCurrent=0  Capacitance=1e-6  Setx0=off  InitialVoltage=0  Measurements=None
  RL2 : powerlib/Elements/Series RLC Branch  LConnTagsString=__new0  RConnTagsString=__new0  BranchType=RL  Resistance=R  Inductance=L  SetiL0=off  InitialCurrent=0  Capacitance=1e-6  Setx0=off  InitialVoltage=0  Measurements=None
  a_in : PMIOPort  Port=1  Side=Left
  a_out : PMIOPort  Port=2  Side=Right
  b_in : PMIOPort  Port=3  Side=Left
  b_out : PMIOPort  Port=4  Side=Right
  connections:
  b_in/RConn1 -- RL2/LConn1
  a_in/RConn1 -- RL1/LConn1
  a_out/RConn1 -- RL1/RConn1
  b_out/RConn1 -- RL2/RConn1

== system typhoonPatterns/Cable 3PH ==
  RL1 : powerlib/Elements/Series RLC Branch  LConnTagsString=__new0  RConnTagsString=__new0  BranchType=RL  Resistance=R  Inductance=L  SetiL0=off  InitialCurrent=0  Capacitance=1e-6  Setx0=off  InitialVoltage=0  Measurements=None
  RL2 : powerlib/Elements/Series RLC Branch  LConnTagsString=__new0  RConnTagsString=__new0  BranchType=RL  Resistance=R  Inductance=L  SetiL0=off  InitialCurrent=0  Capacitance=1e-6  Setx0=off  InitialVoltage=0  Measurements=None
  RL3 : powerlib/Elements/Series RLC Branch  LConnTagsString=__new0  RConnTagsString=__new0  BranchType=RL  Resistance=R  Inductance=L  SetiL0=off  InitialCurrent=0  Capacitance=1e-6  Setx0=off  InitialVoltage=0  Measurements=None
  a_in : PMIOPort  Port=1  Side=Left
  a_out : PMIOPort  Port=2  Side=Right
  b_in : PMIOPort  Port=3  Side=Left
  b_out : PMIOPort  Port=4  Side=Right
  c_in : PMIOPort  Port=5  Side=Left
  c_out : PMIOPort  Port=6  Side=Right
  connections:
  b_out/RConn1 -- RL2/RConn1
  a_out/RConn1 -- RL1/RConn1
  a_in/RConn1 -- RL1/LConn1
  b_in/RConn1 -- RL2/LConn1
  c_in/RConn1 -- RL3/LConn1
  c_out/RConn1 -- RL3/RConn1

== system typhoonPatterns/DC Machine ==
  mech : Inport
  DC Machine1 : powerlib/Machines/DC Machine  PresetModel=No  MechanicalLoad=Torque TL  FieldType=Wound  ShowDetailedParameters=on  MeasurementBus=off  RLa="[Ra_DC  La_DC]"  RLf="[Rf_DC  Lf_DC]"  Laf=Laf_DC  MachineConstant=Torque constant (N.m/A)  Ke=1.8  Kt=1.8  J=Jm  Bm=fc  Tf=0  w0=0  Ifinit=0  TsPowergui=0  TsBlock=-1
  A : PMIOPort  Port=1  Side=Left
  A- : PMIOPort  Port=2  Side=Right
  F+ : PMIOPort  Port=3  Side=Left
  F- : PMIOPort  Port=4  Side=Right
  meas : Outport
  wires:
  mech/1 -> DC Machine1/1
  DC Machine1/1 -> meas/1
  connections:
  A/RConn1 -- DC Machine1/LConn1
  DC Machine1/LConn2 -- F+/RConn1
  DC Machine1/RConn1 -- A-/RConn1
  DC Machine1/RConn2 -- F-/RConn1

== system typhoonPatterns/DPDT Contactor ==
  control : Inport
  Sa_1 : powerlib/Power Electronics/Ideal Switch  Ron=r_on  Lon=0  IC=s0  Rs=r_s  Cs=c_s  Measurements=on
  Sa_2 : powerlib/Power Electronics/Ideal Switch  Ron=r_on  Lon=0  IC=s0  Rs=r_s  Cs=c_s  Measurements=on
  Sb_1 : powerlib/Power Electronics/Ideal Switch  Ron=r_on  Lon=0  IC=s0  Rs=r_s  Cs=c_s  Measurements=on
  Sb_2 : powerlib/Power Electronics/Ideal Switch  Ron=r_on  Lon=0  IC=s0  Rs=r_s  Cs=c_s  Measurements=on
  inv1 : Logic  Commented=through  Operator=NOT  AllPortsSameDT=off  OutDataTypeStr=boolean
  inv2 : Logic  Operator=NOT  AllPortsSameDT=off  OutDataTypeStr=boolean
  A1 : PMIOPort  Port=1  Side=Left
  B1 : PMIOPort  Port=2  Side=Left
  C1 : PMIOPort  Port=3  Side=Right
  A2 : PMIOPort  Port=4  Side=Left
  B2 : PMIOPort  Port=5  Side=Left
  C2 : PMIOPort  Port=6  Side=Right
  wires:
  [S_2] -> Sa_2/1
  [S_1] -> Sa_1/1
  inv2/1 -> [S_2]
  control/1 -> inv1/1
  inv1/1 -> [S_1], inv2/1
  [S_2] -> Sb_2/1
  [S_1] -> Sb_1/1
  connections:
  Sa_1/RConn1 -- C1/RConn1 -- Sa_2/RConn1
  B1/RConn1 -- Sa_2/LConn1
  A1/RConn1 -- Sa_1/LConn1
  Sb_2/RConn1 -- Sb_1/RConn1 -- C2/RConn1
  A2/RConn1 -- Sb_1/LConn1
  B2/RConn1 -- Sb_2/LConn1

== system typhoonPatterns/DPST Contactor ==
  control : Inport
  Sa : powerlib/Power Electronics/Ideal Switch  Ron=r_on  Lon=0  IC=s0  Rs=r_s  Cs=c_s  Measurements=on
  Sb : powerlib/Power Electronics/Ideal Switch  Ron=r_on  Lon=0  IC=s0  Rs=r_s  Cs=c_s  Measurements=on
  inv1 : Logic  Commented=through  Operator=NOT  AllPortsSameDT=off  OutDataTypeStr=boolean
  A1 : PMIOPort  Port=1  Side=Left
  B1 : PMIOPort  Port=2  Side=Right
  A2 : PMIOPort  Port=3  Side=Left
  B2 : PMIOPort  Port=4  Side=Right
  wires:
  [S] -> Sb/1
  inv1/1 -> [S]
  control/1 -> inv1/1
  [S] -> Sa/1
  connections:
  A2/RConn1 -- Sb/LConn1
  B2/RConn1 -- Sb/RConn1
  A1/RConn1 -- Sa/LConn1
  B1/RConn1 -- Sa/RConn1

== system typhoonPatterns/Diode Leg ==
  Bus Creator : BusCreator  Inputs=2
  Bus Creator1 : BusCreator  Inputs=2
  D1 : powerlib/Power Electronics/Diode  Ron=r_on  Lon=0  Vf=v_f  IC=0  UseSnubber=0  Rs=r_s  Cs=c_s  Measurements=on
  D2 : powerlib/Power Electronics/Diode  Ron=r_on  Lon=0  Vf=v_f  IC=0  UseSnubber=0  Rs=r_s  Cs=c_s  Measurements=on
  Demux1 : Demux  Outputs=2
  Demux2 : Demux  Outputs=2
  Selector_i : BusSelector  OutputSignals=i(D1)  OutputAsBus=on
  Selector_v : BusSelector  OutputSignals=v(D1)  OutputAsBus=on
  DC+ : PMIOPort  Port=1  Side=Left
  DC- : PMIOPort  Port=2  Side=Left
  Phase : PMIOPort  Port=3  Side=Right
  i_meas : Outport
  v_meas : Outport  Port=2
  wires:
  Selector_v/1 -> v_meas/1
  Bus Creator1/1 -> Selector_v/1
  [v_S1] -> Bus Creator1/1  "v(D1)"
  [m_S1] -> Demux1/1
  [v_S2] -> Bus Creator1/2  "v(D2)"
  [i_S1] -> Bus Creator/1  "i(D1)"
  [i_S2] -> Bus Creator/2  "i(D2)"
  Selector_i/1 -> i_meas/1
  [m_S2] -> Demux2/1
  Demux2/1 -> [i_S2]
  Demux2/2 -> [v_S2]
  Demux1/2 -> [v_S1]
  Demux1/1 -> [i_S1]
  Bus Creator/1 -> Selector_i/1
  D1/1 -> [m_S1]
  D2/1 -> [m_S2]
  connections:
  D2/LConn1 -- DC-/RConn1
  Phase/RConn1 -- D2/RConn1 -- D1/LConn1
  D1/RConn1 -- DC+/RConn1

== system typhoonPatterns/Diode Rectifier (1-Phase) ==
  Bus Creator : BusCreator  Inputs=4
  Bus Creator1 : BusCreator  Inputs=4
  Demux{1..3,5} (4 alike) : Demux  Outputs=2
  Selector_i : BusSelector  OutputSignals=i(Sa_top)  OutputAsBus=on
  Selector_v : BusSelector  OutputSignals=v(Sa_top)  OutputAsBus=on
  sa_bot : powerlib/Power Electronics/Diode  Ron=r_on  Lon=0  Vf=v_f  IC=0  UseSnubber=0  Rs=r_s  Cs=c_s  Measurements=on
  sa_top : powerlib/Power Electronics/Diode  Ron=r_on  Lon=0  Vf=v_f  IC=0  UseSnubber=0  Rs=r_s  Cs=c_s  Measurements=on
  sb_bot : powerlib/Power Electronics/Diode  Ron=r_on  Lon=0  Vf=v_f  IC=0  UseSnubber=0  Rs=r_s  Cs=c_s  Measurements=on
  sb_top : powerlib/Power Electronics/Diode  Ron=r_on  Lon=0  Vf=v_f  IC=0  UseSnubber=0  Rs=r_s  Cs=c_s  Measurements=on
  A : PMIOPort  Port=1  Side=Left
  B : PMIOPort  Port=2  Side=Left
  DC+ : PMIOPort  Port=3  Side=Right
  DC- : PMIOPort  Port=4  Side=Right
  i_meas : Outport
  v_meas : Outport  Port=2
  wires:
  sa_top/1 -> [m_Sa_top]
  sa_bot/1 -> [m_Sa_bot]
  sb_bot/1 -> [m_Sb_bot]
  sb_top/1 -> [m_Sb_top]
  [m_Sb_top] -> Demux3/1
  Bus Creator/1 -> Selector_i/1
  [m_Sa_bot] -> Demux2/1
  Selector_i/1 -> i_meas/1
  [m_Sa_bot] -> Demux5/1
  [m_Sa_top] -> Demux1/1
  Selector_v/1 -> v_meas/1
  [i_Sa_top] -> Bus Creator/1  "i(Sa_top)"
  Demux1/1 -> [i_Sa_top]
  Demux1/2 -> [v_Sa_top]
  Demux2/1 -> [i_Sa_bot]
  Demux2/2 -> [v_Sa_bot]
  Demux3/1 -> [i_Sb_top]
  Demux5/1 -> [i_Sb_bot]
  Demux5/2 -> [v_Sb_bot]
  Demux3/2 -> [v_Sb_top]
  [i_Sa_bot] -> Bus Creator/2  "i(Sa_bot)"
  [i_Sb_top] -> Bus Creator/3  "i(Sb_top)"
  [i_Sb_bot] -> Bus Creator/4  "i(Sb_bot)"
  [v_Sa_top] -> Bus Creator1/1  "v(Sa_top)"
  [v_Sa_bot] -> Bus Creator1/2  "v(Sa_bot)"
  [v_Sb_top] -> Bus Creator1/3  "v(Sb_top)"
  [v_Sb_bot] -> Bus Creator1/4  "v(Sb_bot)"
  Bus Creator1/1 -> Selector_v/1
  connections:
  sa_top/LConn1 -- sa_bot/RConn1 -- A/RConn1
  sb_top/LConn1 -- sb_bot/RConn1 -- B/RConn1
  sb_top/RConn1 -- DC+/RConn1 -- sa_top/RConn1
  sb_bot/LConn1 -- DC-/RConn1 -- sa_bot/LConn1

== system typhoonPatterns/Diode Rectifier (3-Phase) ==
  Bus Creator1 : BusCreator  Inputs=6
  Bus Creator2 : BusCreator  Inputs=6
  Demux{1..2,4,8..10} (6 alike) : Demux  Outputs=2
  Selector_i : BusSelector  OutputSignals=i(Sa_top)  OutputAsBus=on
  Selector_v : BusSelector  OutputSignals=v(Sa_top)  OutputAsBus=on
  sa_bot : powerlib/Power Electronics/Diode  Ron=r_on  Lon=0  Vf=v_f  IC=0  UseSnubber=0  Rs=r_s  Cs=c_s  Measurements=on
  sa_top : powerlib/Power Electronics/Diode  Ron=r_on  Lon=0  Vf=v_f  IC=0  UseSnubber=0  Rs=r_s  Cs=c_s  Measurements=on
  sb_bot : powerlib/Power Electronics/Diode  Ron=r_on  Lon=0  Vf=v_f  IC=0  UseSnubber=0  Rs=r_s  Cs=c_s  Measurements=on
  sb_top : powerlib/Power Electronics/Diode  Ron=r_on  Lon=0  Vf=v_f  IC=0  UseSnubber=0  Rs=r_s  Cs=c_s  Measurements=on
  sc_bot : powerlib/Power Electronics/Diode  Ron=r_on  Lon=0  Vf=v_f  IC=0  UseSnubber=0  Rs=r_s  Cs=c_s  Measurements=on
  sc_top : powerlib/Power Electronics/Diode  Ron=r_on  Lon=0  Vf=v_f  IC=0  UseSnubber=0  Rs=r_s  Cs=c_s  Measurements=on
  A : PMIOPort  Port=1  Side=Left
  B : PMIOPort  Port=2  Side=Left
  C : PMIOPort  Port=3  Side=Left
  DC+ : PMIOPort  Port=4  Side=Right
  DC- : PMIOPort  Port=5  Side=Right
  i_meas : Outport
  v_meas : Outport  Port=2
  wires:
  sa_top/1 -> [m_Sa_top]
  sa_bot/1 -> [m_Sa_bot]
  sb_bot/1 -> [m_Sb_bot]
  sc_bot/1 -> [m_Sc_bot]
  sc_top/1 -> [m_Sc_top]
  sb_top/1 -> [m_Sb_top]
  Demux8/2 -> [v_Sa_bot]
  Demux4/2 -> [v_Sa_top]
  [v_Sa_top] -> Bus Creator2/1  "v(Sa_top)"
  [i_Sb_top] -> Bus Creator1/3  "i(Sb_top)"
  [i_Sb_bot] -> Bus Creator1/4  "i(Sb_bot)"
  Demux10/2 -> [v_Sb_bot]
  Bus Creator2/1 -> Selector_v/1
  Demux9/2 -> [v_Sb_top]
  [v_Sb_bot] -> Bus Creator2/4  "v(Sb_bot)"
  Demux10/1 -> [i_Sb_bot]
  Selector_v/1 -> v_meas/1
  [v_Sb_top] -> Bus Creator2/3  "v(Sb_top)"
  [m_Sb_bot] -> Demux10/1
  [m_Sa_bot] -> Demux8/1
  Demux4/1 -> [i_Sa_top]
  [m_Sa_top] -> Demux4/1
  Bus Creator1/1 -> Selector_i/1
  [m_Sb_top] -> Demux9/1
  Demux8/1 -> [i_Sa_bot]
  Selector_i/1 -> i_meas/1
  Demux9/1 -> [i_Sb_top]
  [v_Sa_bot] -> Bus Creator2/2  "v(Sa_bot)"
  [i_Sa_bot] -> Bus Creator1/2  "i(Sa_bot)"
  [i_Sa_top] -> Bus Creator1/1  "i(Sa_top)"
  [m_Sc_bot] -> Demux1/1
  Demux1/2 -> [v_Sc_bot]
  Demux2/1 -> [i_Sc_top]
  Demux1/1 -> [i_Sc_bot]
  Demux2/2 -> [v_Sc_top]
  [m_Sc_top] -> Demux2/1
  [i_Sc_top] -> Bus Creator1/5  "i(Sc_top)"
  [i_Sc_bot] -> Bus Creator1/6  "i(Sc_bot)"
  [v_Sc_top] -> Bus Creator2/5  "v(Sc_top)"
  [v_Sc_bot] -> Bus Creator2/6  "v(Sc_bot)"
  connections:
  C/RConn1 -- sc_bot/RConn1 -- sc_top/LConn1
  sc_bot/LConn1 -- sa_bot/LConn1 -- sb_bot/LConn1 -- DC-/RConn1
  sc_top/RConn1 -- sa_top/RConn1 -- sb_top/RConn1 -- DC+/RConn1
  A/RConn1 -- sa_bot/RConn1 -- sa_top/LConn1
  B/RConn1 -- sb_bot/RConn1 -- sb_top/LConn1

== system typhoonPatterns/FC Leg (3-level) ==
  gate : Inport
  Bus Creator1 : BusCreator  Inputs=4
  Bus Creator2 : BusCreator  Inputs=4
  Demux : Demux
  Demux{1..3,6} (4 alike) : Demux  Outputs=2
  S{1..4} (4 alike) : powerlib/Power Electronics/IGBT//Diode  Ron=r_on  Rs=r_s  Cs=c_s  Measurements=on
  Selector_i : BusSelector  OutputSignals=i(S1)  OutputAsBus=on
  Selector_v : BusSelector  OutputSignals=v(S1)  OutputAsBus=on
  inv{1..4} (4 alike) : Logic  Commented=through  Operator=NOT  AllPortsSameDT=off  OutDataTypeStr=boolean
  DC+ : PMIOPort  Port=1  Side=Left
  C1 : PMIOPort  Port=2  Side=Left
  C2 : PMIOPort  Port=3  Side=Left
  DC- : PMIOPort  Port=4  Side=Left
  Phase : PMIOPort  Port=5  Side=Right
  i_meas : Outport
  v_meas : Outport  Port=2
  wires:
  Demux3/1 -> [i_S3]
  Demux/4 -> inv4/1
  Bus Creator2/1 -> Selector_v/1
  inv3/1 -> [S3]
  Demux2/1 -> [i_S4]
  [m_S3] -> Demux3/1
  [i_S3] -> Bus Creator1/3  "i(S3)"
  [i_S2] -> Bus Creator1/2  "i(S2)"
  [S3] -> S3/1
  [m_S1] -> Demux6/1
  S4/1 -> [m_S4]
  Demux6/1 -> [i_S1]
  [i_S4] -> Bus Creator1/4  "i(S4)"
  Demux2/2 -> [v_S4]
  [v_S1] -> Bus Creator2/1  "v(S1)"
  Selector_v/1 -> v_meas/1
  S2/1 -> [m_S2]
  [S2] -> S2/1
  [m_S2] -> Demux1/1
  Demux/3 -> inv3/1
  Selector_i/1 -> i_meas/1
  Bus Creator1/1 -> Selector_i/1
  [m_S4] -> Demux2/1
  inv1/1 -> [S1]
  inv2/1 -> [S2]
  Demux/1 -> inv1/1
  inv4/1 -> [S4]
  S3/1 -> [m_S3]
  [i_S1] -> Bus Creator1/1  "i(S1)"
  Demux/2 -> inv2/1
  Demux6/2 -> [v_S1]
  [v_S2] -> Bus Creator2/2  "v(S2)"
  Demux3/2 -> [v_S3]
  gate/1 -> Demux/1
  [v_S4] -> Bus Creator2/4  "v(S4)"
  Demux1/1 -> [i_S2]
  S1/1 -> [m_S1]
  [S1] -> S1/1
  [v_S3] -> Bus Creator2/3  "v(S3)"
  [S4] -> S4/1
  Demux1/2 -> [v_S2]
  connections:
  S3/LConn1 -- Phase/RConn1 -- S2/RConn1
  S1/RConn1 -- S2/LConn1 -- C1/RConn1
  S4/LConn1 -- C2/RConn1 -- S3/RConn1
  S1/LConn1 -- DC+/RConn1
  DC-/RConn1 -- S4/RConn1

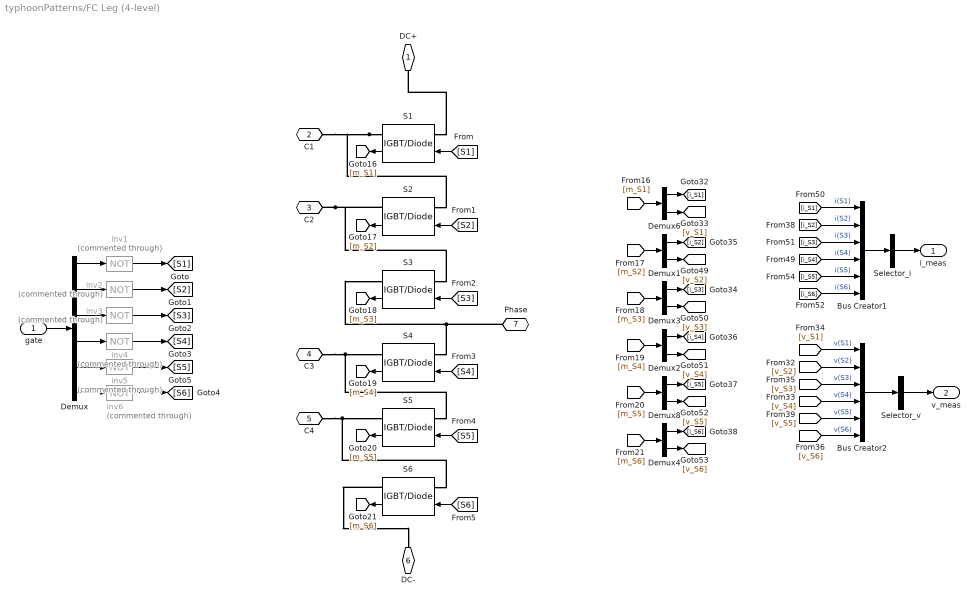
== system typhoonPatterns/FC Leg (4-level) ==
  gate : Inport
  Bus Creator1 : BusCreator  Inputs=6
  Bus Creator2 : BusCreator  Inputs=6
  Demux : Demux  Outputs=6
  Demux{1..4,6,8} (6 alike) : Demux  Outputs=2
  S{1..6} (6 alike) : powerlib/Power Electronics/IGBT//Diode  Ron=r_on  Rs=r_s  Cs=c_s  Measurements=on
  Selector_i : BusSelector  OutputSignals=i(S1)  OutputAsBus=on
  Selector_v : BusSelector  OutputSignals=v(S1)  OutputAsBus=on
  inv{1..6} (6 alike) : Logic  Commented=through  Operator=NOT  AllPortsSameDT=off  OutDataTypeStr=boolean
  DC+ : PMIOPort  Port=1  Side=Left
  C1 : PMIOPort  Port=2  Side=Left
  C2 : PMIOPort  Port=3  Side=Left
  C3 : PMIOPort  Port=4  Side=Left
  C4 : PMIOPort  Port=5  Side=Left
  DC- : PMIOPort  Port=6  Side=Left
  Phase : PMIOPort  Port=7  Side=Right
  i_meas : Outport
  v_meas : Outport  Port=2
  wires:
  inv1/1 -> [S1]
  inv4/1 -> [S4]
  S3/1 -> [m_S3]
  Demux8/2 -> [v_S5]
  Demux/1 -> inv1/1
  S1/1 -> [m_S1]
  Selector_i/1 -> i_meas/1
  Demux/3 -> inv3/1
  [S6] -> S6/1
  inv6/1 -> [S6]
  [S5] -> S5/1
  [S2] -> S2/1
  S2/1 -> [m_S2]
  [m_S4] -> Demux2/1
  [i_S6] -> Bus Creator1/6  "i(S6)"
  Demux/5 -> inv5/1
  S6/1 -> [m_S6]
  inv5/1 -> [S5]
  [m_S2] -> Demux1/1
  [v_S1] -> Bus Creator2/1  "v(S1)"
  Demux4/2 -> [v_S6]
  Demux/6 -> inv6/1
  Demux2/2 -> [v_S4]
  Demux6/1 -> [i_S1]
  [i_S4] -> Bus Creator1/4  "i(S4)"
  [m_S1] -> Demux6/1
  [i_S2] -> Bus Creator1/2  "i(S2)"
  [i_S3] -> Bus Creator1/3  "i(S3)"
  [i_S5] -> Bus Creator1/5  "i(S5)"
  Demux8/1 -> [i_S5]
  gate/1 -> Demux/1
  [m_S3] -> Demux3/1
  [S3] -> S3/1
  S5/1 -> [m_S5]
  Selector_v/1 -> v_meas/1
  [m_S5] -> Demux8/1
  S4/1 -> [m_S4]
  [v_S2] -> Bus Creator2/2  "v(S2)"
  [m_S6] -> Demux4/1
  Bus Creator2/1 -> Selector_v/1
  Demux2/1 -> [i_S4]
  inv3/1 -> [S3]
  Demux/2 -> inv2/1
  Bus Creator1/1 -> Selector_i/1
  Demux/4 -> inv4/1
  Demux4/1 -> [i_S6]
  [v_S6] -> Bus Creator2/6  "v(S6)"
  [v_S3] -> Bus Creator2/3  "v(S3)"
  Demux3/2 -> [v_S3]
  Demux6/2 -> [v_S1]
  [S1] -> S1/1
  [i_S1] -> Bus Creator1/1  "i(S1)"
  [v_S4] -> Bus Creator2/4  "v(S4)"
  Demux1/1 -> [i_S2]
  [S4] -> S4/1
  inv2/1 -> [S2]
  [v_S5] -> Bus Creator2/5  "v(S5)"
  Demux1/2 -> [v_S2]
  Demux3/1 -> [i_S3]
  connections:
  S4/LConn1 -- S3/RConn1 -- Phase/RConn1
  C2/RConn1 -- S2/RConn1 -- S3/LConn1
  S1/RConn1 -- S2/LConn1 -- C1/RConn1
  S6/RConn1 -- DC-/RConn1
  S6/LConn1 -- S5/RConn1 -- C4/RConn1
  S5/LConn1 -- S4/RConn1 -- C3/RConn1
  S1/LConn1 -- DC+/RConn1

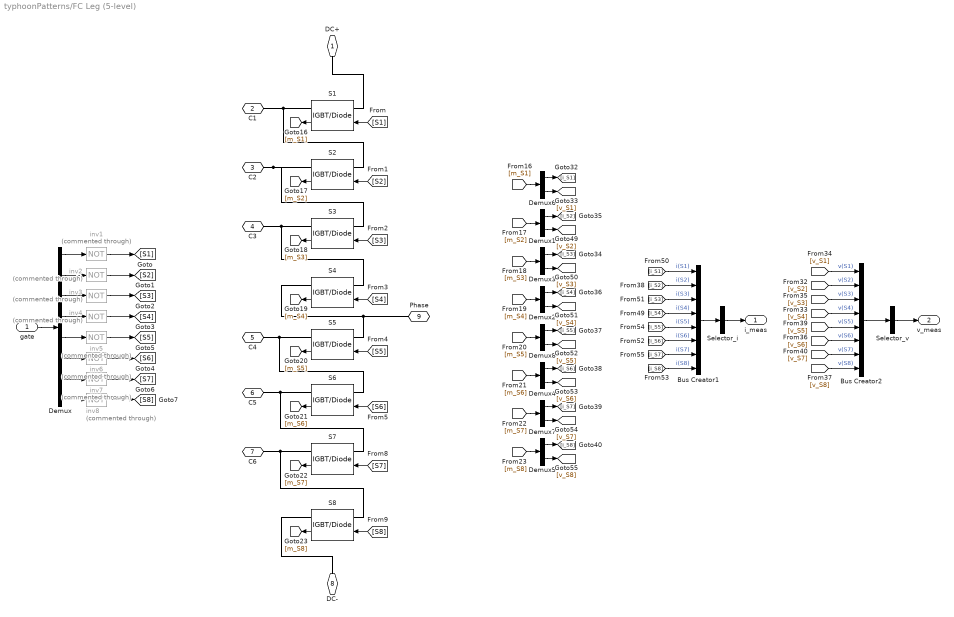
== system typhoonPatterns/FC Leg (5-level) ==
  gate : Inport
  Bus Creator1 : BusCreator  Inputs=8
  Bus Creator2 : BusCreator  Inputs=8
  Demux : Demux  Outputs=8
  Demux{1..8} (8 alike) : Demux  Outputs=2
  S{1..8} (8 alike) : powerlib/Power Electronics/IGBT//Diode  Ron=r_on  Rs=r_s  Cs=c_s  Measurements=on
  Selector_i : BusSelector  OutputSignals=i(S1)  OutputAsBus=on
  Selector_v : BusSelector  OutputSignals=v(S1)  OutputAsBus=on
  inv{1..8} (8 alike) : Logic  Commented=through  Operator=NOT  AllPortsSameDT=off  OutDataTypeStr=boolean
  DC+ : PMIOPort  Port=1  Side=Left
  C1 : PMIOPort  Port=2  Side=Left
  C2 : PMIOPort  Port=3  Side=Left
  C3 : PMIOPort  Port=4  Side=Left
  C4 : PMIOPort  Port=5  Side=Left
  C5 : PMIOPort  Port=6  Side=Left
  C6 : PMIOPort  Port=7  Side=Left
  DC- : PMIOPort  Port=8  Side=Left
  Phase : PMIOPort  Port=9  Side=Right
  i_meas : Outport
  v_meas : Outport  Port=2
  wires:
  [S3] -> S3/1
  Demux7/2 -> [v_S7]
  Demux8/2 -> [v_S5]
  S3/1 -> [m_S3]
  inv4/1 -> [S4]
  inv1/1 -> [S1]
  [S1] -> S1/1
  [S8] -> S8/1
  inv5/1 -> [S5]
  [m_S2] -> Demux1/1
  S6/1 -> [m_S6]
  [m_S4] -> Demux2/1
  S7/1 -> [m_S7]
  [m_S7] -> Demux7/1
  [m_S1] -> Demux6/1
  Demux1/2 -> [v_S2]
  Demux/7 -> inv7/1
  S4/1 -> [m_S4]
  [S4] -> S4/1
  Demux/5 -> inv5/1
  Demux/8 -> inv8/1
  [v_S5] -> Bus Creator2/5  "v(S5)"
  [S2] -> S2/1
  [i_S6] -> Bus Creator1/6  "i(S6)"
  [i_S8] -> Bus Creator1/8  "i(S8)"
  Demux3/1 -> [i_S3]
  [S7] -> S7/1
  [S5] -> S5/1
  Demux/3 -> inv3/1
  [S6] -> S6/1
  S8/1 -> [m_S8]
  inv8/1 -> [S8]
  inv6/1 -> [S6]
  Demux8/1 -> [i_S5]
  [m_S8] -> Demux5/1
  S1/1 -> [m_S1]
  Selector_i/1 -> i_meas/1
  Demux4/2 -> [v_S6]
  S2/1 -> [m_S2]
  Demux/1 -> inv1/1
  [v_S4] -> Bus Creator2/4  "v(S4)"
  S5/1 -> [m_S5]
  [m_S3] -> Demux3/1
  Demux/4 -> inv4/1
  Demux7/1 -> [i_S7]
  Demux4/1 -> [i_S6]
  gate/1 -> Demux/1
  [i_S3] -> Bus Creator1/3  "i(S3)"
  [i_S5] -> Bus Creator1/5  "i(S5)"
  [i_S1] -> Bus Creator1/1  "i(S1)"
  [m_S5] -> Demux8/1
  [i_S4] -> Bus Creator1/4  "i(S4)"
  [i_S2] -> Bus Creator1/2  "i(S2)"
  [i_S7] -> Bus Creator1/7  "i(S7)"
  Bus Creator2/1 -> Selector_v/1
  Demux6/1 -> [i_S1]
  Demux/6 -> inv6/1
  [v_S1] -> Bus Creator2/1  "v(S1)"
  Demux6/2 -> [v_S1]
  [v_S8] -> Bus Creator2/8  "v(S8)"
  Demux2/2 -> [v_S4]
  Demux3/2 -> [v_S3]
  [v_S7] -> Bus Creator2/7  "v(S7)"
  Demux1/1 -> [i_S2]
  inv7/1 -> [S7]
  [v_S6] -> Bus Creator2/6  "v(S6)"
  [v_S3] -> Bus Creator2/3  "v(S3)"
  Bus Creator1/1 -> Selector_i/1
  Demux2/1 -> [i_S4]
  inv3/1 -> [S3]
  Demux/2 -> inv2/1
  [v_S2] -> Bus Creator2/2  "v(S2)"
  Demux5/1 -> [i_S8]
  Demux5/2 -> [v_S8]
  [m_S6] -> Demux4/1
  Selector_v/1 -> v_meas/1
  inv2/1 -> [S2]
  connections:
  C1/RConn1 -- S2/LConn1 -- S1/RConn1
  S8/LConn1 -- S7/RConn1 -- C6/RConn1
  S5/LConn1 -- S4/RConn1 -- Phase/RConn1
  C3/RConn1 -- S4/LConn1 -- S3/RConn1
  S6/LConn1 -- C4/RConn1 -- S5/RConn1
  C2/RConn1 -- S2/RConn1 -- S3/LConn1
  S7/LConn1 -- C5/RConn1 -- S6/RConn1
  S1/LConn1 -- DC+/RConn1
  DC-/RConn1 -- S8/RConn1
